simulink model "NPC_inverter_nfE_TS_203864"  (R2023b)
settings: Solver=ode4  StartTime=0.0  StopTime=Tsim  FixedStep=Ts  RelTol=1e-3
InitFcn:
  | run('param_nfE.m');
values from neighbouring files (symbols this model uses):
  f = 50    [param_nfE.m]
  KI = (1/K2)*(1-zR1)*(1-zR1)    [param_nfE.m]
  KP = (1/K2)*(1+K1-2*zR1)    [param_nfE.m]
  LN = 1e-3    (= 0.001)    [param_nfE.m]
  M = (1/K2)*(1-zR1)    [param_nfE.m]
  mmax = 1    [param_nfE.m]
  mmin = -1    [param_nfE.m]
  TA = Tc    (= 0.000125)    [param_nfE.m]
  Tc = 1/fc    (= 0.000125)    [param_nfE.m]
  Umax = Ud/2    (= 350)    [param_nfE.m]
undefined symbols (not defined in the file or in its folder): plecs
libraries: simulink x12, plecslib x5
settings Model: Creator=timsp  LastModifiedBy=timsp

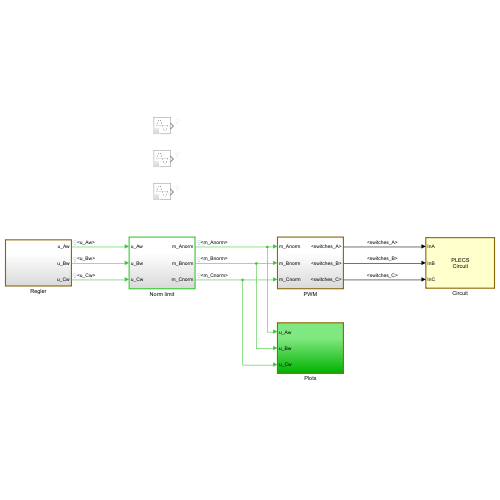
[thumbnail: Simulink's stored preview of the top-level diagram]
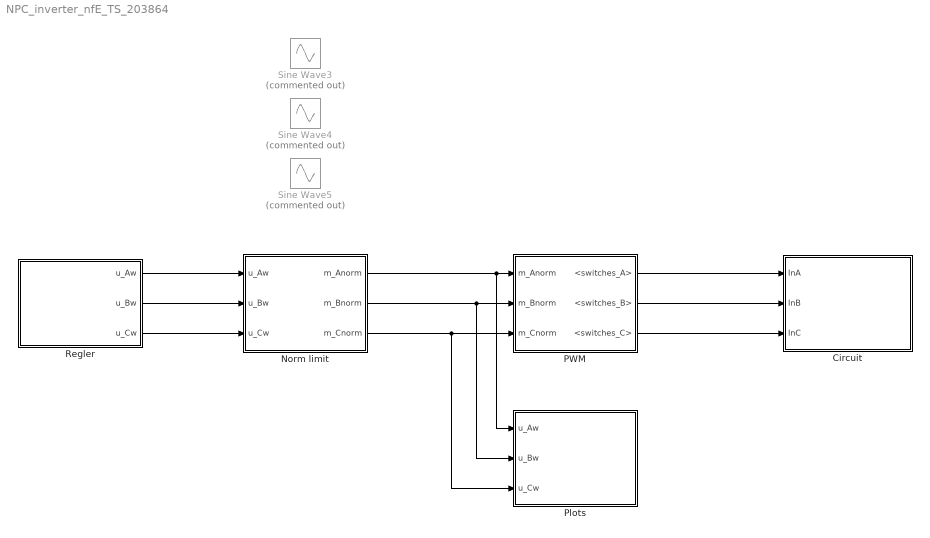
== system NPC_inverter_nfE_TS_203864 ==
  Circuit : Subsystem  LoadFcn=plecs('sl', 200);  InitFcn=plecs('sl', 214);  StartFcn=plecs('sl', 208);  StopFcn=plecs('sl', 209);  mask(PlecsCircuit){PLECSData=<binary blob, 5092 chars, not shown>}
      mask prompts: PLECSData "PLECS Data (Do not delete or modify!)"
      mask init:
      | % PLACE CUSTOM INITIALIZATIONS ABOVE
      | % DO NOT REMOVE
      | plecs('sl', 215);
      | % DO NOT REMOVE
      settings: CopyFcn=plecs('sl', 203);  DeleteFcn=plecs('sl', 205);  UndoDeleteFcn=plecs('sl', 206);  PreSaveFcn=plecs('sl', 211);  PostSaveFcn=plecs('sl', 201);  NameChangeFcn=plecs('sl', 210);  DestroyFcn=plecs('sl', 207);  PreCopyFcn=plecs('sl', 216);  OpenFcn=plecs('sl', 202);  ErrorFcn=plerrorfcn
      mask Help: eval('plecs(''help'', ''qthelp:///creatingacircuit.html'')')
      mask Display: disp('PLECS\nCircuit')
  Norm limit : Subsystem
  PWM : Subsystem
  Plots : Subsystem
  Regler : Subsystem
  Sine Wave3 : Sin  Commented=on  Amplitude=sqrt(2)*230  Frequency=2*pi*f  SampleTime=0
  Sine Wave4 : Sin  Commented=on  Amplitude=sqrt(2)*230  Frequency=2*pi*f  Phase=-2*pi/3  SampleTime=0
  Sine Wave5 : Sin  Commented=on  Amplitude=sqrt(2)*230  Frequency=2*pi*f  Phase=-4*pi/3  SampleTime=0
  wires:
  PWM/1(<switches_A>) -> Circuit/1(InA)
  PWM/2(<switches_B>) -> Circuit/2(InB)
  PWM/3(<switches_C>) -> Circuit/3(InC)
  Norm limit/1(m_Anorm) -> Plots/1(u_Aw), PWM/1(m_Anorm)
  Norm limit/2(m_Bnorm) -> PWM/2(m_Bnorm), Plots/2(u_Bw)
  Norm limit/3(m_Cnorm) -> PWM/3(m_Cnorm), Plots/3(u_Cw)
  Regler/1(u_Aw) -> Norm limit/1(u_Aw)
  Regler/2(u_Bw) -> Norm limit/2(u_Bw)
  Regler/3(u_Cw) -> Norm limit/3(u_Cw)

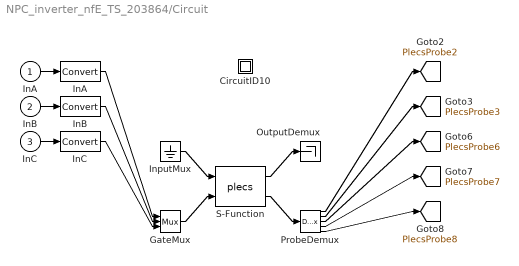
== system NPC_inverter_nfE_TS_203864/Circuit ==
  InA : Inport  PortDimensions=4
  InB : Inport  Port=2  PortDimensions=4
  InC : Inport  Port=3  PortDimensions=4
  " CircuitID10 " : Subsystem
  " GateMux " : Mux  Inputs=[ 4 4 4 ]
  " InA " : DataTypeConversion
  " InB " : DataTypeConversion
  " InC " : DataTypeConversion
  " InputMux " : Ground
  " OutputDemux " : Terminator
  " ProbeDemux " : Demux  Outputs=[ 3 3 3 3 3 ]
  " S-Function " : S-Function  FunctionName=plecs  SFunctionDeploymentMode=off  EnableBusSupport=off
  tag scope: PlecsProbe2=global, PlecsProbe3=global, PlecsProbe6=global, PlecsProbe7=global, PlecsProbe8=global
  wires:
  " InputMux "/1 -> " S-Function "/1
  " GateMux "/1 -> " S-Function "/2
  " S-Function "/1 -> " OutputDemux "/1
  " S-Function "/2 -> " ProbeDemux "/1
  InA/1 -> " InA "/1
  " InA "/1 -> " GateMux "/1
  InB/1 -> " InB "/1
  " InB "/1 -> " GateMux "/2
  InC/1 -> " InC "/1
  " InC "/1 -> " GateMux "/3
  " ProbeDemux "/1 -> [PlecsProbe2]
  " ProbeDemux "/2 -> [PlecsProbe3]
  " ProbeDemux "/3 -> [PlecsProbe6]
  " ProbeDemux "/4 -> [PlecsProbe7]
  " ProbeDemux "/5 -> [PlecsProbe8]

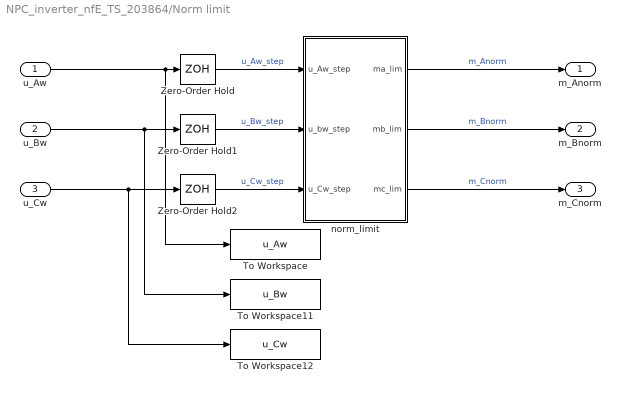
== system NPC_inverter_nfE_TS_203864/Norm limit ==
  u_Aw : Inport
  u_Bw : Inport  Port=2
  u_Cw : Inport  Port=3
  To Workspace : ToWorkspace  VariableName=u_Aw  SampleTime=-1
      settings: Save2DSignal=2-D array (concatenate along first dimension)
  To Workspace11 : ToWorkspace  VariableName=u_Bw  SampleTime=-1
      settings: Save2DSignal=2-D array (concatenate along first dimension)
  To Workspace12 : ToWorkspace  VariableName=u_Cw  SampleTime=-1
      settings: Save2DSignal=2-D array (concatenate along first dimension)
  Zero-Order Hold : ZeroOrderHold  SampleTime=TA
  Zero-Order Hold1 : ZeroOrderHold  SampleTime=TA
  Zero-Order Hold2 : ZeroOrderHold  SampleTime=TA
  norm_limit : Subsystem
  m_Anorm : Outport
  m_Bnorm : Outport  Port=2
  m_Cnorm : Outport  Port=3
  wires:
  norm_limit/2(mb_lim) -> m_Bnorm/1  "m_Bnorm"
  u_Aw/1 -> Zero-Order Hold/1, To Workspace/1
  norm_limit/3(mc_lim) -> m_Cnorm/1  "m_Cnorm"
  Zero-Order Hold1/1 -> norm_limit/2(u_bw_step)  "u_Bw_step"
  u_Bw/1 -> Zero-Order Hold1/1, To Workspace11/1
  Zero-Order Hold/1 -> norm_limit/1(u_Aw_step)  "u_Aw_step"
  u_Cw/1 -> Zero-Order Hold2/1, To Workspace12/1
  Zero-Order Hold2/1 -> norm_limit/3(u_Cw_step)  "u_Cw_step"
  norm_limit/1(ma_lim) -> m_Anorm/1  "m_Anorm"

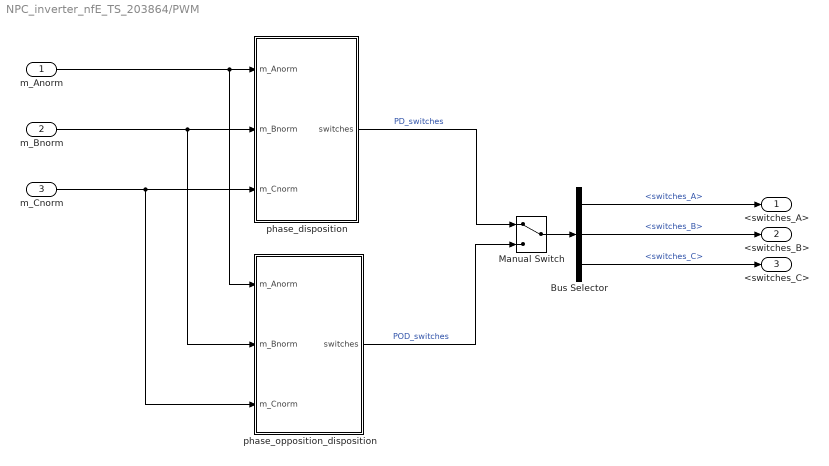
== system NPC_inverter_nfE_TS_203864/PWM ==
  m_Anorm : Inport
  m_Bnorm : Inport  Port=2
  m_Cnorm : Inport  Port=3
  Bus Selector : BusSelector  OutputSignals=switches_A,switches_B,switches_C
  Manual Switch : ManualSwitch
  phase_disposition : Subsystem  TreatAsAtomicUnit=on
  phase_opposition_disposition : Subsystem  TreatAsAtomicUnit=on
  <switches_A> : Outport
  <switches_B> : Outport  Port=2
  <switches_C> : Outport  Port=3
  wires:
  Bus Selector/1 -> <switches_A>/1  "<switches_A>"
  phase_disposition/1(switches) -> Manual Switch/1  "PD_switches"
  Bus Selector/3 -> <switches_C>/1  "<switches_C>"
  phase_opposition_disposition/1(switches) -> Manual Switch/2  "POD_switches"
  Manual Switch/1 -> Bus Selector/1
  Bus Selector/2 -> <switches_B>/1  "<switches_B>"
  m_Anorm/1 -> phase_opposition_disposition/1(m_Anorm), phase_disposition/1(m_Anorm)
  m_Cnorm/1 -> phase_opposition_disposition/3(m_Cnorm), phase_disposition/3(m_Cnorm)
  m_Bnorm/1 -> phase_opposition_disposition/2(m_Bnorm), phase_disposition/2(m_Bnorm)

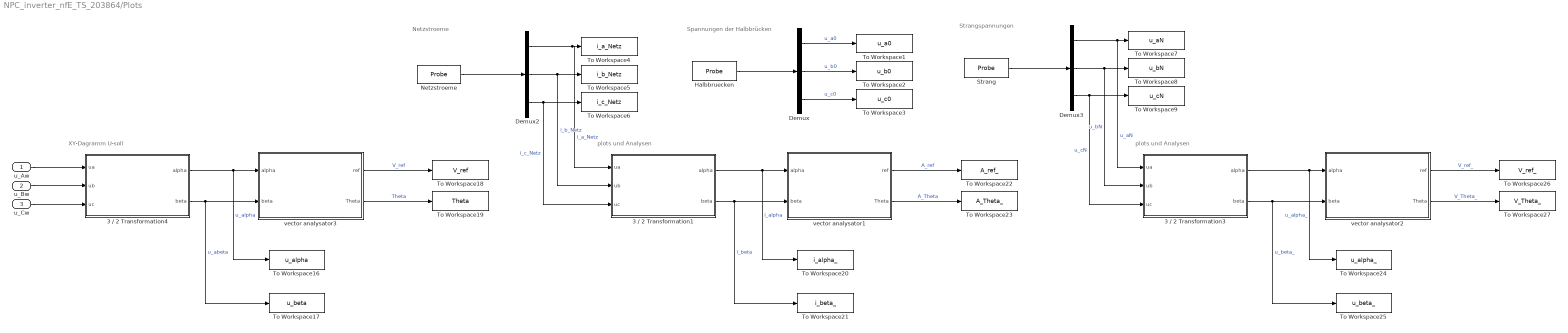
== system NPC_inverter_nfE_TS_203864/Plots ==
  note: Spannungen der Halbbrücken
  note: Strangspannungen
  note: Netzstroeme
  note: plots und Analysen
  note: plots und Analysen
  note: XY-Dagramm U-soll
  u_Aw : Inport
  u_Bw : Inport  Port=2
  u_Cw : Inport  Port=3
  3 / 2 Transformation1 : MATLAB Function  TreatAsAtomicUnit=on
  3 / 2 Transformation3 : MATLAB Function  TreatAsAtomicUnit=on
  3 / 2 Transformation4 : MATLAB Function  TreatAsAtomicUnit=on
  Demux : Demux  Outputs=3
  Demux2 : Demux  Outputs=3
  Demux3 : Demux  Outputs=3
  Halbbruecken : plecslib/Probe  tagno=2
      settings: SourceProductName=PLECS
  Netzstroeme : plecslib/Probe  tagno=8
      settings: SourceProductName=PLECS
  Strang : plecslib/Probe  tagno=3
      settings: SourceProductName=PLECS
  To Workspace1 : ToWorkspace  VariableName=u_a0  SampleTime=-1
  To Workspace16 : ToWorkspace  VariableName=u_alpha  SampleTime=-1
  To Workspace17 : ToWorkspace  VariableName=u_beta  SampleTime=-1
  To Workspace18 : ToWorkspace  VariableName=V_ref  SampleTime=-1
  To Workspace19 : ToWorkspace  VariableName=Theta  SampleTime=-1
  To Workspace2 : ToWorkspace  VariableName=u_b0  SampleTime=-1
  To Workspace20 : ToWorkspace  VariableName=i_alpha_  SampleTime=-1
  To Workspace21 : ToWorkspace  VariableName=i_beta_  SampleTime=-1
  To Workspace22 : ToWorkspace  VariableName=A_ref_  SampleTime=-1
  To Workspace23 : ToWorkspace  VariableName=A_Theta_  SampleTime=-1
  To Workspace24 : ToWorkspace  VariableName=u_alpha_  SampleTime=-1
  To Workspace25 : ToWorkspace  VariableName=u_beta_  SampleTime=-1
  To Workspace26 : ToWorkspace  VariableName=V_ref_  SampleTime=-1
  To Workspace27 : ToWorkspace  VariableName=V_Theta_  SampleTime=-1
  To Workspace3 : ToWorkspace  VariableName=u_c0  SampleTime=-1
  To Workspace4 : ToWorkspace  VariableName=i_a_Netz  SampleTime=-1
  To Workspace5 : ToWorkspace  VariableName=i_b_Netz  SampleTime=-1
  To Workspace6 : ToWorkspace  VariableName=i_c_Netz  SampleTime=-1
  To Workspace7 : ToWorkspace  VariableName=u_aN  SampleTime=-1
  To Workspace8 : ToWorkspace  VariableName=u_bN  SampleTime=-1
  To Workspace9 : ToWorkspace  VariableName=u_cN  SampleTime=-1
  vector analysator1 : MATLAB Function  TreatAsAtomicUnit=on
  vector analysator2 : MATLAB Function  TreatAsAtomicUnit=on
  vector analysator3 : MATLAB Function  TreatAsAtomicUnit=on
  wires:
  Demux2/2 -> To Workspace5/1, 3 / 2 Transformation1/2(ub)  "i_b_Netz"
  Netzstroeme/1 -> Demux2/1
  Demux/3 -> To Workspace3/1  "u_c0"
  3 / 2 Transformation1/2(beta) -> To Workspace21/1, vector analysator1/2(beta)  "i_beta"
  vector analysator2/1(ref) -> To Workspace26/1  "V_ref_"
  3 / 2 Transformation1/1(alpha) -> To Workspace20/1, vector analysator1/1(alpha)  "i_alpha"
  Demux2/1 -> 3 / 2 Transformation1/1(ua), To Workspace4/1  "i_a_Netz"
  3 / 2 Transformation3/2(beta) -> To Workspace25/1, vector analysator2/2(beta)  "u_beta_"
  vector analysator1/2(Theta) -> To Workspace23/1  "A_Theta"
  vector analysator2/2(Theta) -> To Workspace27/1  "V_Theta_"
  3 / 2 Transformation3/1(alpha) -> To Workspace24/1, vector analysator2/1(alpha)  "u_alpha_"
  vector analysator1/1(ref) -> To Workspace22/1  "A_ref"
  Halbbruecken/1 -> Demux/1
  Demux3/1 -> To Workspace7/1, 3 / 2 Transformation3/1(ua)  "u_aN"
  Demux2/3 -> To Workspace6/1, 3 / 2 Transformation1/3(uc)  "i_c_Netz"
  Demux3/3 -> To Workspace9/1, 3 / 2 Transformation3/3(uc)  "u_cN"
  Demux3/2 -> To Workspace8/1, 3 / 2 Transformation3/2(ub)  "u_bN"
  Demux/1 -> To Workspace1/1  "u_a0"
  Strang/1 -> Demux3/1
  Demux/2 -> To Workspace2/1  "u_b0"
  u_Aw/1 -> 3 / 2 Transformation4/1(ua)
  vector analysator3/1(ref) -> To Workspace18/1  "V_ref"
  u_Bw/1 -> 3 / 2 Transformation4/2(ub)
  3 / 2 Transformation4/2(beta) -> To Workspace17/1, vector analysator3/2(beta)  "u_abeta"
  u_Cw/1 -> 3 / 2 Transformation4/3(uc)
  3 / 2 Transformation4/1(alpha) -> To Workspace16/1, vector analysator3/1(alpha)  "u_alpha"
  vector analysator3/2(Theta) -> To Workspace19/1  "Theta"

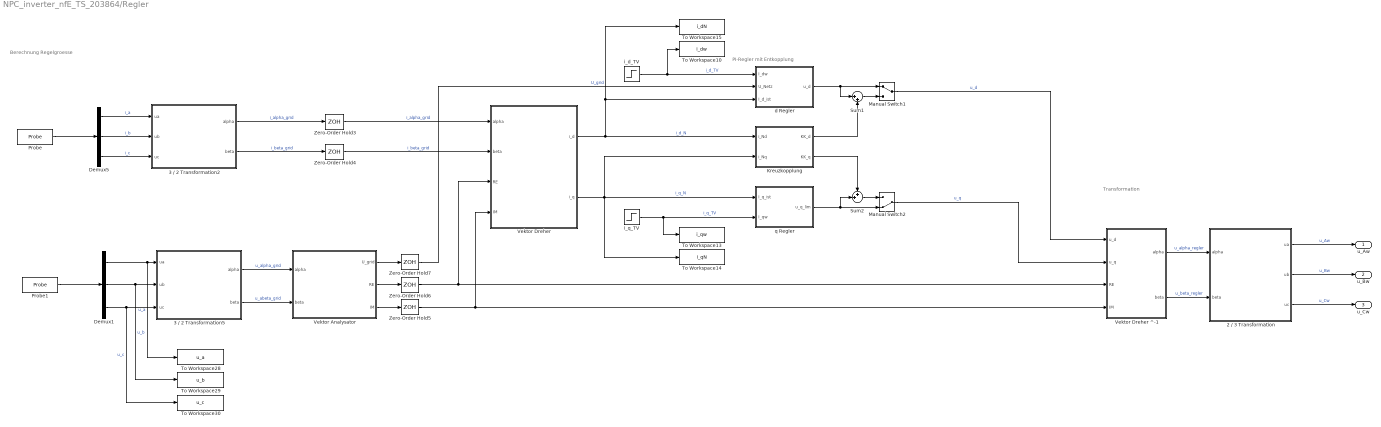
== system NPC_inverter_nfE_TS_203864/Regler ==
  note: Transformation
  note: PI-Regler mit Entkopplung
  note: Berechnung Regelgroesse
  "2 / 3 Transformation " : MATLAB Function  TreatAsAtomicUnit=on
  3 / 2 Transformation2 : MATLAB Function  TreatAsAtomicUnit=on
  3 / 2 Transformation5 : MATLAB Function  TreatAsAtomicUnit=on
  Demux1 : Demux  Outputs=3
  Demux5 : Demux  Outputs=3
  Kreuzkopplung : Subsystem
  Manual Switch1 : ManualSwitch
  Manual Switch2 : ManualSwitch  CurrentSetting=0
  Probe : plecslib/Probe  tagno=6
      settings: SourceProductName=PLECS
  Probe1 : plecslib/Probe  tagno=7
      settings: SourceProductName=PLECS
  Sum1 : Sum  Inputs=|++
  Sum2 : Sum  Inputs=++|
  To Workspace10 : ToWorkspace  VariableName=i_dw  SampleTime=-1
  To Workspace13 : ToWorkspace  VariableName=i_qw  SampleTime=-1
  To Workspace14 : ToWorkspace  VariableName=i_qN  SampleTime=-1
  To Workspace15 : ToWorkspace  VariableName=i_dN  SampleTime=-1
  To Workspace28 : ToWorkspace  VariableName=u_a  SampleTime=-1
  To Workspace29 : ToWorkspace  VariableName=u_b  SampleTime=-1
  To Workspace30 : ToWorkspace  VariableName=u_c  SampleTime=-1
  Vektor Analysator : MATLAB Function  TreatAsAtomicUnit=on
  Vektor Dreher : MATLAB Function  TreatAsAtomicUnit=on
  Vektor Dreher ^-1 : MATLAB Function  TreatAsAtomicUnit=on
  Zero-Order Hold{3..7} (5 alike) : ZeroOrderHold  SampleTime=TA
  d Regler : Subsystem  TreatAsAtomicUnit=on  SystemSampleTime=TA
  i_d_TV : Step  Time=0.025  Before=20  After=-20  SampleTime=TA
  i_q_TV : Step  Time=0.05  After=20  SampleTime=TA
  q Regler : Subsystem  TreatAsAtomicUnit=on  SystemSampleTime=TA
  u_Aw : Outport
  u_Bw : Outport  Port=2
  u_Cw : Outport  Port=3
  wires:
  Vektor Analysator/1(U_grid) -> Zero-Order Hold7/1
  Vektor Dreher/2(i_q) -> Kreuzkopplung/2(i_Nq), q Regler/1(I_q_ist), To Workspace14/1  "i_q_N"
  Vektor Analysator/3(IM) -> Zero-Order Hold5/1
  i_d_TV/1 -> To Workspace10/1, d Regler/1(I_dw)  "i_d_TV"
  Zero-Order Hold4/1 -> Vektor Dreher/2(beta)  "i_beta_grid"
  Zero-Order Hold3/1 -> Vektor Dreher/1(alpha)  "i_alpha_grid"
  Vektor Dreher/1(i_d) -> d Regler/3(I_d_ist), To Workspace15/1, Kreuzkopplung/1(i_Nd)  "i_d_N"
  Probe1/1 -> Demux1/1
  q Regler/1(u_q_lim) -> Manual Switch2/2, Sum2/2
  Manual Switch1/1 -> Vektor Dreher ^-1/1(u_d)  "u_d"
  Sum2/1 -> Manual Switch2/1
  Demux1/1 -> To Workspace28/1, 3 / 2 Transformation5/1(ua)  "u_a"
  Probe/1 -> Demux5/1
  "2 / 3 Transformation "/1(ua) -> u_Aw/1  "u_Aw"
  "2 / 3 Transformation "/3(uc) -> u_Cw/1  "u_Cw"
  3 / 2 Transformation2/2(beta) -> Zero-Order Hold4/1  "i_beta_grid"
  Demux5/1 -> 3 / 2 Transformation2/1(ua)  "i_a"
  i_q_TV/1 -> q Regler/2(I_qw), To Workspace13/1  "i_q_TV"
  Kreuzkopplung/1(KK_d) -> Sum1/2
  Kreuzkopplung/2(KK_q) -> Sum2/1
  Zero-Order Hold5/1 -> Vektor Dreher/4(IM), Vektor Dreher ^-1/4(IM)
  Demux5/2 -> 3 / 2 Transformation2/2(ub)  "i_b"
  Sum1/1 -> Manual Switch1/2
  Zero-Order Hold6/1 -> Vektor Dreher ^-1/3(RE), Vektor Dreher/3(RE)
  Manual Switch2/1 -> Vektor Dreher ^-1/2(u_q)  "u_q"
  Demux5/3 -> 3 / 2 Transformation2/3(uc)  "i_c"
  Vektor Analysator/2(RE) -> Zero-Order Hold6/1
  d Regler/1(u_d) -> Manual Switch1/1, Sum1/1
  Demux1/3 -> To Workspace30/1, 3 / 2 Transformation5/3(uc)  "u_c"
  3 / 2 Transformation2/1(alpha) -> Zero-Order Hold3/1  "i_alpha_grid"
  3 / 2 Transformation5/1(alpha) -> Vektor Analysator/1(alpha)  "u_alpha_grid"
  Demux1/2 -> To Workspace29/1, 3 / 2 Transformation5/2(ub)  "u_b"
  Vektor Dreher ^-1/2(beta) -> "2 / 3 Transformation "/2(beta)  "u_beta_regler"
  3 / 2 Transformation5/2(beta) -> Vektor Analysator/2(beta)  "u_abeta_grid"
  "2 / 3 Transformation "/2(ub) -> u_Bw/1  "u_Bw"
  Zero-Order Hold7/1 -> d Regler/2(U_Netz)  "U_grid"
  Vektor Dreher ^-1/1(alpha) -> "2 / 3 Transformation "/1(alpha)  "u_alpha_regler"

== system NPC_inverter_nfE_TS_203864/Circuit/ CircuitID10  ==

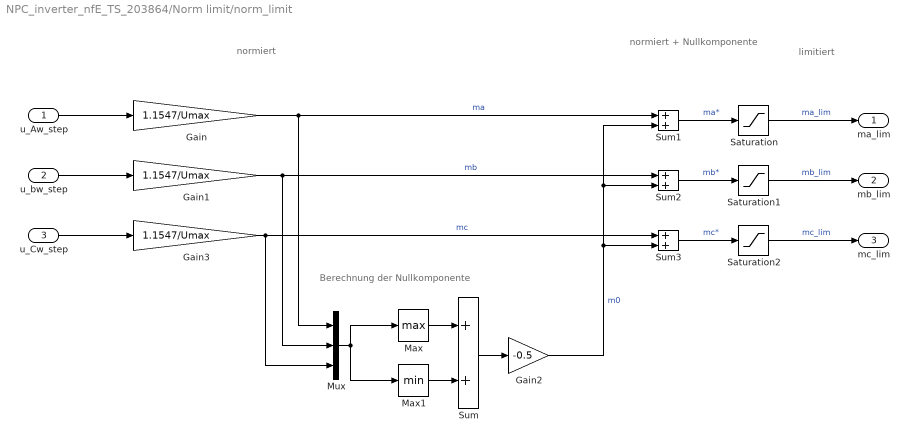
== system NPC_inverter_nfE_TS_203864/Norm limit/norm_limit ==
  note: limitiert
  note: normiert
      | + Nullkomponente
  note: normiert
  note: Berechnung der Nullkomponente
  u_Aw_step : Inport
  u_bw_step : Inport  Port=2
  u_Cw_step : Inport  Port=3
  Gain : Gain  Gain=1.1547/Umax
  Gain1 : Gain  Gain=1.1547/Umax
  Gain2 : Gain  Gain=-0.5
  Gain3 : Gain  Gain=1.1547/Umax
  Max : MinMax  Function=max
  Max1 : MinMax
  Mux : Mux  Inputs=3
  Saturation : Saturate  UpperLimit=mmax  LowerLimit=mmin
  Saturation1 : Saturate  UpperLimit=mmax  LowerLimit=mmin
  Saturation2 : Saturate  UpperLimit=mmax  LowerLimit=mmin
  Sum{,1..3} (4 alike) : Sum
  ma_lim : Outport
  mb_lim : Outport  Port=2
  mc_lim : Outport  Port=3
  wires:
  Gain2/1 -> Sum1/2, Sum2/2, Sum3/2  "m0"
  Sum3/1 -> Saturation2/1  "mc*"
  Sum2/1 -> Saturation1/1  "mb*"
  Sum1/1 -> Saturation/1  "ma*"
  Gain/1 -> Mux/1, Sum1/1  "ma"
  Mux/1 -> Max/1, Max1/1
  Gain1/1 -> Sum2/1, Mux/2  "mb"
  Max1/1 -> Sum/2
  Sum/1 -> Gain2/1
  Max/1 -> Sum/1
  Gain3/1 -> Mux/3, Sum3/1  "mc"
  Saturation2/1 -> mc_lim/1  "mc_lim"
  Saturation1/1 -> mb_lim/1  "mb_lim"
  Saturation/1 -> ma_lim/1  "ma_lim"
  u_Aw_step/1 -> Gain/1
  u_bw_step/1 -> Gain1/1
  u_Cw_step/1 -> Gain3/1

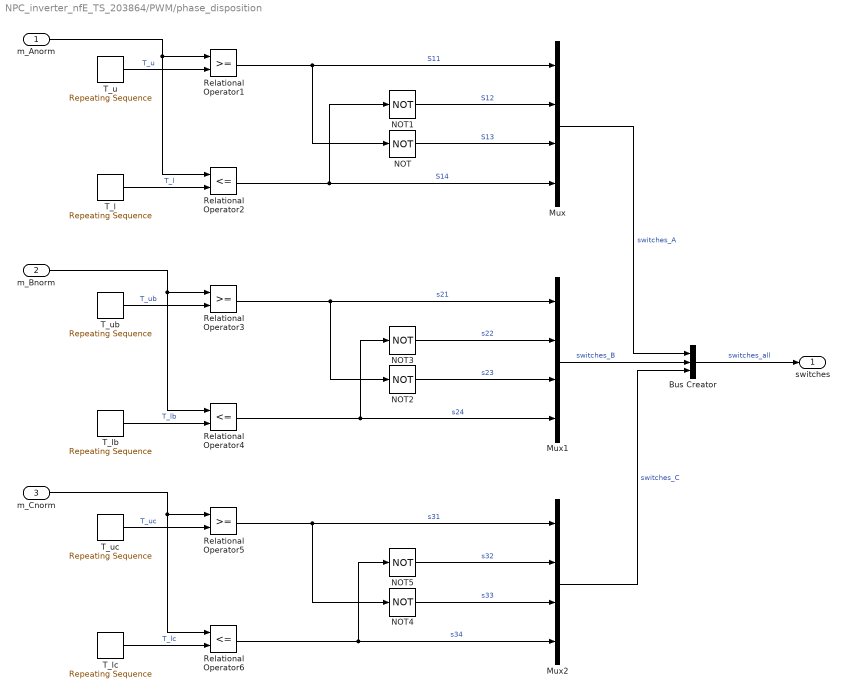
== system NPC_inverter_nfE_TS_203864/PWM/phase_disposition ==
  m_Anorm : Inport
  m_Bnorm : Inport  Port=2
  m_Cnorm : Inport  Port=3
  Bus Creator : BusCreator  Inputs=3
  Mux : Mux
  Mux1 : Mux
  Mux2 : Mux
  NOT{,1..5} (6 alike) : Logic  Operator=NOT  AllPortsSameDT=off  OutDataTypeStr=boolean
  Relational Operator1 : RelationalOperator  OutDataTypeStr=boolean  RndMeth=Simplest  InputSameDT=off
  Relational Operator2 : RelationalOperator  Operator=<=  OutDataTypeStr=boolean  RndMeth=Simplest  InputSameDT=off
  Relational Operator3 : RelationalOperator  OutDataTypeStr=boolean  RndMeth=Simplest  InputSameDT=off
  Relational Operator4 : RelationalOperator  Operator=<=  OutDataTypeStr=boolean  RndMeth=Simplest  InputSameDT=off
  Relational Operator5 : RelationalOperator  OutDataTypeStr=boolean  RndMeth=Simplest  InputSameDT=off
  Relational Operator6 : RelationalOperator  Operator=<=  OutDataTypeStr=boolean  RndMeth=Simplest  InputSameDT=off
  T_l : simulink/Sources/Repeating Sequence  rep_seq_t=[0 Tc/2 Tc]  rep_seq_y=[-1 0 -1]
  T_lb : simulink/Sources/Repeating Sequence  rep_seq_t=[0 Tc/2 Tc]  rep_seq_y=[-1 0 -1]
  T_lc : simulink/Sources/Repeating Sequence  rep_seq_t=[0 Tc/2 Tc]  rep_seq_y=[-1 0 -1]
  T_u : simulink/Sources/Repeating Sequence  rep_seq_t=[0 Tc/2 Tc]  rep_seq_y=[0 1 0]
  T_ub : simulink/Sources/Repeating Sequence  rep_seq_t=[0 Tc/2 Tc]  rep_seq_y=[0 1 0]
  T_uc : simulink/Sources/Repeating Sequence  rep_seq_t=[0 Tc/2 Tc]  rep_seq_y=[0 1 0]
  switches : Outport
  wires:
  Bus Creator/1 -> switches/1  "switches_all"
  m_Anorm/1 -> Relational Operator2/1, Relational Operator1/1
  Relational Operator1/1 -> NOT/1, Mux/1  "S11"
  Relational Operator2/1 -> NOT1/1, Mux/4  "S14"
  T_l/1 -> Relational Operator2/2  "T_l"
  T_u/1 -> Relational Operator1/2  "T_u"
  NOT/1 -> Mux/3  "S13"
  NOT1/1 -> Mux/2  "S12"
  NOT2/1 -> Mux1/3  "s23"
  NOT3/1 -> Mux1/2  "s22"
  T_lb/1 -> Relational Operator4/2  "T_lb"
  Relational Operator3/1 -> NOT2/1, Mux1/1  "s21"
  Relational Operator4/1 -> Mux1/4, NOT3/1  "s24"
  T_ub/1 -> Relational Operator3/2  "T_ub"
  T_uc/1 -> Relational Operator5/2  "T_uc"
  Relational Operator6/1 -> Mux2/4, NOT5/1  "s34"
  T_lc/1 -> Relational Operator6/2  "T_lc"
  NOT4/1 -> Mux2/3  "s33"
  Relational Operator5/1 -> NOT4/1, Mux2/1  "s31"
  NOT5/1 -> Mux2/2  "s32"
  Mux/1 -> Bus Creator/1  "switches_A"
  Mux1/1 -> Bus Creator/2  "switches_B"
  Mux2/1 -> Bus Creator/3  "switches_C"
  m_Cnorm/1 -> Relational Operator6/1, Relational Operator5/1
  m_Bnorm/1 -> Relational Operator4/1, Relational Operator3/1

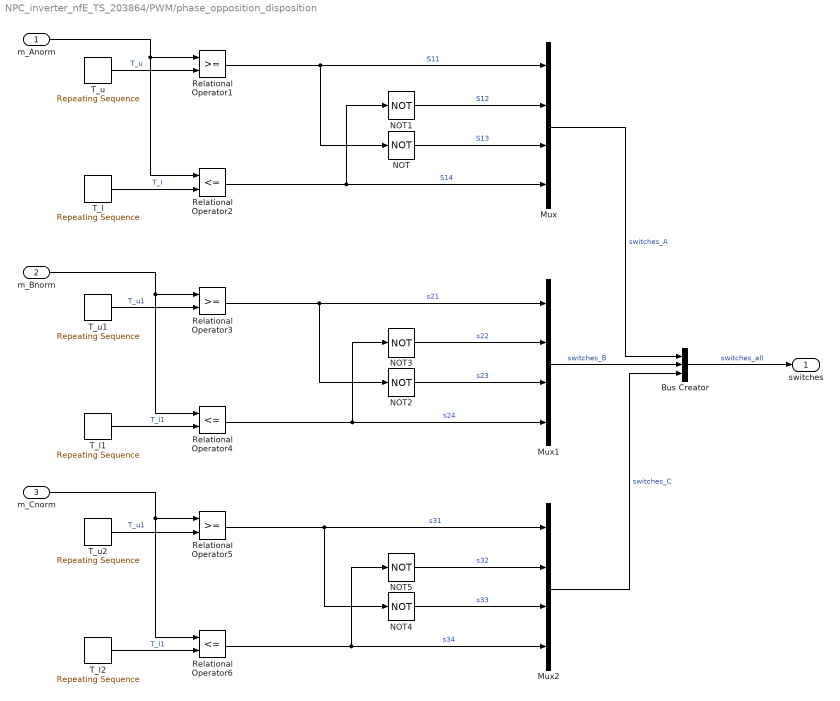
== system NPC_inverter_nfE_TS_203864/PWM/phase_opposition_disposition ==
  m_Anorm : Inport
  m_Bnorm : Inport  Port=2
  m_Cnorm : Inport  Port=3
  Bus Creator : BusCreator  Inputs=3
  Mux : Mux
  Mux1 : Mux
  Mux2 : Mux
  NOT{,1..5} (6 alike) : Logic  Operator=NOT  AllPortsSameDT=off  OutDataTypeStr=boolean
  Relational Operator1 : RelationalOperator  OutDataTypeStr=boolean  RndMeth=Simplest  InputSameDT=off
  Relational Operator2 : RelationalOperator  Operator=<=  OutDataTypeStr=boolean  RndMeth=Simplest  InputSameDT=off
  Relational Operator3 : RelationalOperator  OutDataTypeStr=boolean  RndMeth=Simplest  InputSameDT=off
  Relational Operator4 : RelationalOperator  Operator=<=  OutDataTypeStr=boolean  RndMeth=Simplest  InputSameDT=off
  Relational Operator5 : RelationalOperator  OutDataTypeStr=boolean  RndMeth=Simplest  InputSameDT=off
  Relational Operator6 : RelationalOperator  Operator=<=  OutDataTypeStr=boolean  RndMeth=Simplest  InputSameDT=off
  T_l : simulink/Sources/Repeating Sequence  rep_seq_t=[0 Tc/2 Tc]  rep_seq_y=[ 0 -1 0]
  T_l1 : simulink/Sources/Repeating Sequence  rep_seq_t=[0 Tc/2 Tc]  rep_seq_y=[0 -1 0]
  T_l2 : simulink/Sources/Repeating Sequence  rep_seq_t=[0 Tc/2 Tc]  rep_seq_y=[0 -1 0]
  T_u : simulink/Sources/Repeating Sequence  rep_seq_t=[0 Tc/2 Tc]  rep_seq_y=[0 1 0]
  T_u1 : simulink/Sources/Repeating Sequence  rep_seq_t=[0 Tc/2 Tc]  rep_seq_y=[0 1 0]
  T_u2 : simulink/Sources/Repeating Sequence  rep_seq_t=[0 Tc/2 Tc]  rep_seq_y=[0 1 0]
  switches : Outport
  wires:
  Relational Operator6/1 -> NOT5/1, Mux2/4  "s34"
  Bus Creator/1 -> switches/1  "switches_all"
  Relational Operator3/1 -> NOT2/1, Mux1/1  "s21"
  m_Anorm/1 -> Relational Operator2/1, Relational Operator1/1
  T_u/1 -> Relational Operator1/2  "T_u"
  T_l/1 -> Relational Operator2/2  "T_l"
  NOT2/1 -> Mux1/3  "s23"
  Relational Operator1/1 -> Mux/1, NOT/1  "S11"
  Relational Operator2/1 -> Mux/4, NOT1/1  "S14"
  NOT1/1 -> Mux/2  "S12"
  Mux2/1 -> Bus Creator/3  "switches_C"
  NOT3/1 -> Mux1/2  "s22"
  NOT4/1 -> Mux2/3  "s33"
  m_Bnorm/1 -> Relational Operator4/1, Relational Operator3/1
  NOT5/1 -> Mux2/2  "s32"
  T_u2/1 -> Relational Operator5/2  "T_u1"
  Mux1/1 -> Bus Creator/2  "switches_B"
  NOT/1 -> Mux/3  "S13"
  Relational Operator4/1 -> NOT3/1, Mux1/4  "s24"
  Relational Operator5/1 -> Mux2/1, NOT4/1  "s31"
  T_u1/1 -> Relational Operator3/2  "T_u1"
  Mux/1 -> Bus Creator/1  "switches_A"
  T_l1/1 -> Relational Operator4/2  "T_l1"
  m_Cnorm/1 -> Relational Operator6/1, Relational Operator5/1
  T_l2/1 -> Relational Operator6/2  "T_l1"

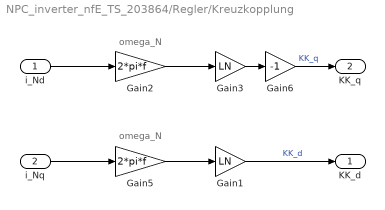
== system NPC_inverter_nfE_TS_203864/Regler/Kreuzkopplung ==
  note: omega_N
  note: omega_N
  i_Nd : Inport
  i_Nq : Inport  Port=2
  Gain1 : Gain  Gain=LN
  Gain2 : Gain  Gain=2*pi*f
  Gain3 : Gain  Gain=LN
  Gain5 : Gain  Gain=2*pi*f
  Gain6 : Gain  Gain=-1
  KK_d : Outport
  KK_q : Outport  Port=2
  wires:
  Gain1/1 -> KK_d/1  "KK_d"
  Gain3/1 -> Gain6/1
  Gain2/1 -> Gain3/1
  i_Nd/1 -> Gain2/1
  Gain5/1 -> Gain1/1
  i_Nq/1 -> Gain5/1
  Gain6/1 -> KK_q/1  "KK_q"

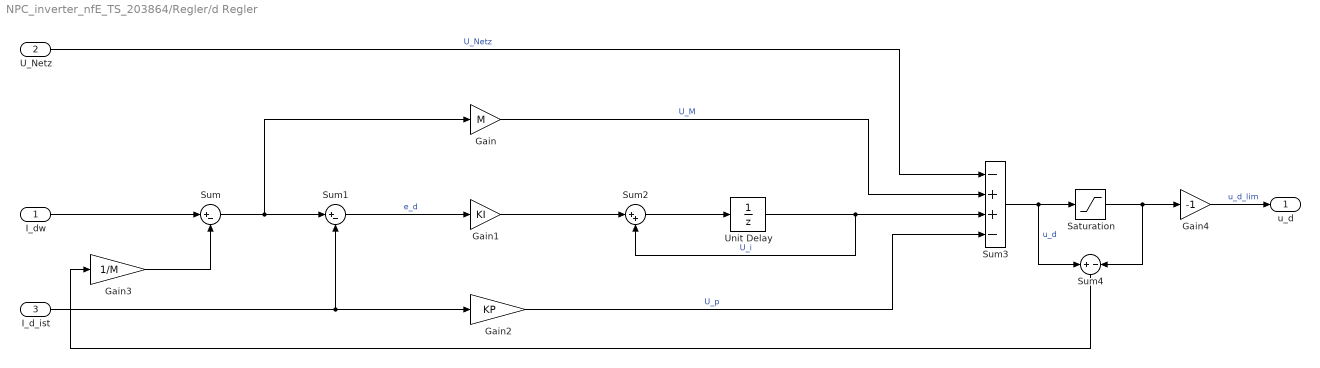
== system NPC_inverter_nfE_TS_203864/Regler/d Regler ==
  I_dw : Inport
  U_Netz : Inport  Port=2
  I_d_ist : Inport  Port=3
  Gain : Gain  Gain=M
  Gain1 : Gain  Gain=KI
  Gain2 : Gain  Gain=KP
  Gain3 : Gain  Gain=1/M
  Gain4 : Gain  Gain=-1
  Saturation : Saturate  UpperLimit=mmax*Umax  LowerLimit=mmin*Umax
  Sum : Sum  Inputs=|+-
  Sum1 : Sum  Inputs=|+-
  Sum2 : Sum  Inputs=|++
  Sum3 : Sum  Inputs=-++-
  Sum4 : Sum  Inputs=+|-
  Unit Delay : UnitDelay  SampleTime=TA  HasFrameUpgradeWarning=on
  u_d : Outport
  wires:
  U_Netz/1 -> Sum3/1  "U_Netz"
  Sum4/1 -> Gain3/1
  Gain3/1 -> Sum/2
  Gain2/1 -> Sum3/4  "U_p"
  Gain/1 -> Sum3/2  "U_M"
  Sum3/1 -> Saturation/1, Sum4/1  "u_d"
  Saturation/1 -> Gain4/1, Sum4/2
  Unit Delay/1 -> Sum3/3, Sum2/2  "U_i"
  Sum2/1 -> Unit Delay/1
  Gain1/1 -> Sum2/1
  Sum1/1 -> Gain1/1  "e_d"
  Sum/1 -> Sum1/1, Gain/1
  I_d_ist/1 -> Sum1/2, Gain2/1
  I_dw/1 -> Sum/1
  Gain4/1 -> u_d/1  "u_d_lim"

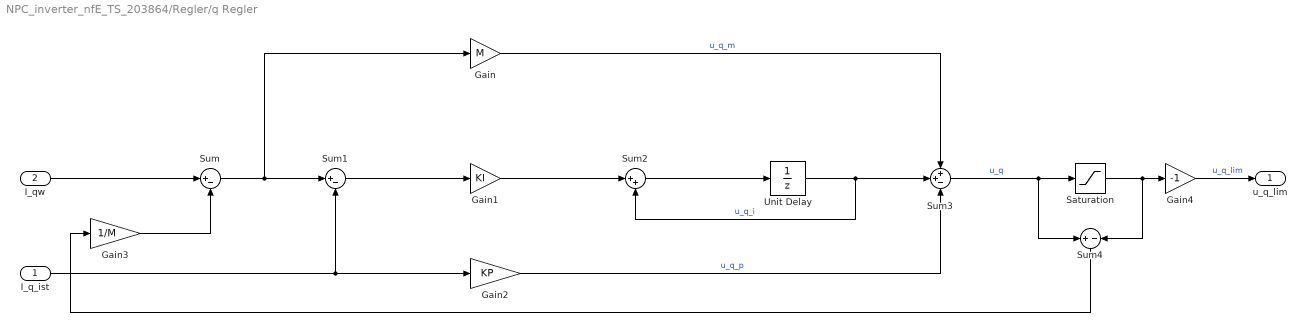
== system NPC_inverter_nfE_TS_203864/Regler/q Regler ==
  I_q_ist : Inport
  I_qw : Inport  Port=2
  Gain : Gain  Gain=M
  Gain1 : Gain  Gain=KI
  Gain2 : Gain  Gain=KP
  Gain3 : Gain  Gain=1/M
  Gain4 : Gain  Gain=-1
  Saturation : Saturate  UpperLimit=mmax*Umax  LowerLimit=mmin*Umax
  Sum : Sum  Inputs=|+-
  Sum1 : Sum  Inputs=|+-
  Sum2 : Sum  Inputs=|++
  Sum3 : Sum  Inputs=++-
  Sum4 : Sum  Inputs=+|-
  Unit Delay : UnitDelay  SampleTime=TA  HasFrameUpgradeWarning=on
  u_q_lim : Outport
  wires:
  Sum/1 -> Sum1/1, Gain/1
  Sum2/1 -> Unit Delay/1
  Gain/1 -> Sum3/1  "u_q_m"
  Gain3/1 -> Sum/2
  Saturation/1 -> Gain4/1, Sum4/2
  I_q_ist/1 -> Sum1/2, Gain2/1
  I_qw/1 -> Sum/1
  Gain1/1 -> Sum2/1
  Gain2/1 -> Sum3/3  "u_q_p"
  Unit Delay/1 -> Sum2/2, Sum3/2  "u_q_i"
  Sum4/1 -> Gain3/1
  Sum3/1 -> Saturation/1, Sum4/1  "u_q"
  Sum1/1 -> Gain1/1
  Gain4/1 -> u_q_lim/1  "u_q_lim"

== matlab function NPC_inverter_nfE_TS_203864/Regler/Vektor Analysator ==
  data: U_grid output; RE output; IM output; alpha input; beta input
function [U_grid, RE, IM]= fcn(alpha, beta)


    U_grid = sqrt(alpha^2+beta^2);

    %Theta = atan2(beta, alpha); % damit Theta [0, 2pi]

    RE = alpha/U_grid;
    
    IM = beta/U_grid;

end

== matlab function NPC_inverter_nfE_TS_203864/Regler/Vektor Dreher ==
  data: alpha input; i_d output; beta input; RE input; IM input; i_q output
function [i_d, i_q]= fcn(alpha, beta, RE, IM)


    
    z = [alpha; beta];

    T =[RE IM ;...
        -IM RE];

    y = T * z;    % [i_alpha ; i_beta]

    i_d = y(1);
    i_q = y(2);

end

== matlab function NPC_inverter_nfE_TS_203864/Regler/Vektor Dreher ^-1 ==
  data: u_d input; alpha output; u_q input; RE input; IM input; beta output
function [alpha, beta] = fcn(u_d, u_q, RE, IM)
    
    z = [u_d;u_q];

    T =[RE -IM ;...
        IM RE];

    y = T * z;    % [alpha; beta]
    
    alpha = y(1);
    beta = y(2);
    %out_0 = 0;

end

== matlab function NPC_inverter_nfE_TS_203864/Plots/vector analysator3 ==
  data: alpha input; ref output; Theta output; beta input
function [ref, Theta]= fcn(alpha, beta)
% ### input vector ###
% u1 = alpha (real part or space vector)
% u2 = beta (imaginary part of space vector)

% ### output vector ###
% y1 = ref (absolute value)
% y2 = Theta (angle)

% ### calculation ####
    ref = sqrt(alpha^2+beta^2);

    Theta = atan2(beta, alpha); % damit Theta [0, 2pi]

end

== matlab function NPC_inverter_nfE_TS_203864/Plots/3 // 2 Transformation1 ==
  data: ua input; alpha output; ub input; uc input; beta output
function [alpha, beta] = fcn(ua, ub, uc)
% ### input vector ###
% u1 = ua
% u2 = ub
% u3 = uc

% ### output vector ###
% y1 = alpha
% y2 = beta
% y3 = u_0

% ### calculation ###
    T = 2/3.*   [1 -1/2 -1/2;...
                0 sqrt(3)/2 -sqrt(3)/2;...
                1/2 1/2 1/2];
    
    y = T * [ua; ub; uc];   
    
% ### return ###
    alpha = y(1);
    beta = y(2);
    %u_0 = y(3);
end

== matlab function NPC_inverter_nfE_TS_203864/Plots/vector analysator1 ==
  data: alpha input; ref output; Theta output; beta input
function [ref, Theta]= fcn(alpha, beta)
% ### input vector ###
% u1 = alpha (real part or space vector)
% u2 = beta (imaginary part of space vector)

% ### output vector ###
% y1 = ref (absolute value)
% y2 = Theta (angle)

% ### calculation ####
    ref = sqrt(alpha^2+beta^2);

    Theta = atan2(beta, alpha); % damit Theta [0, 2pi]

end

== matlab function NPC_inverter_nfE_TS_203864/Plots/3 // 2 Transformation3 ==
  data: ua input; alpha output; ub input; uc input; beta output
function [alpha, beta] = fcn(ua, ub, uc)
% ### input vector ###
% u1 = ua
% u2 = ub
% u3 = uc

% ### output vector ###
% y1 = alpha
% y2 = beta
% y3 = u_0

% ### calculation ###
    T = 2/3.*   [1 -1/2 -1/2;...
                0 sqrt(3)/2 -sqrt(3)/2;...
                1/2 1/2 1/2];
    
    y = T * [ua; ub; uc];   
    
% ### return ###
    alpha = y(1);
    beta = y(2);
    %u_0 = y(3);
end

== matlab function NPC_inverter_nfE_TS_203864/Plots/3 // 2 Transformation4 ==
  data: ua input; alpha output; ub input; uc input; beta output
function [alpha, beta] = fcn(ua, ub, uc)
% ### input vector ###
% u1 = ua
% u2 = ub
% u3 = uc

% ### output vector ###
% y1 = alpha
% y2 = beta
% y3 = u_0

% ### calculation ###
    T = 2/3.*   [1 -1/2 -1/2;...
                0 sqrt(3)/2 -sqrt(3)/2;...
                1/2 1/2 1/2];
    
    y = T * [ua; ub; uc];   
    
% ### return ###
    alpha = y(1);
    beta = y(2);
    %u_0 = y(3);
end

== matlab function NPC_inverter_nfE_TS_203864/Plots/vector analysator2 ==
  data: alpha input; ref output; Theta output; beta input
function [ref, Theta]= fcn(alpha, beta)
% ### input vector ###
% u1 = alpha (real part or space vector)
% u2 = beta (imaginary part of space vector)

% ### output vector ###
% y1 = ref (absolute value)
% y2 = Theta (angle)

% ### calculation ####
    ref = sqrt(alpha^2+beta^2);

    Theta = atan2(beta, alpha); % damit Theta [0, 2pi]

end

== matlab function NPC_inverter_nfE_TS_203864/Regler/2 // 3 Transformation  ==
  data: alpha input; ua output; beta input; ub output; uc output
function [ua, ub, uc] = fcn(alpha, beta)
% ### input vector ###
% y1 = alpha
% y2 = beta
% y3 = u_0 --> no actual input

% ### output vector ###
% u1 = ua
% u2 = ub
% u3 = uc

% ### calculation ###

    T =    [1      0         1;...
           -1/2  sqrt(3)/2   1;...
           -1/2 -sqrt(3)/2   1];
    
    y = T * [alpha; beta; 0];   

% ### return ###
    ua = y(1);
    ub = y(2);
    uc = y(3);
end

== matlab function NPC_inverter_nfE_TS_203864/Regler/3 // 2 Transformation2 ==
  data: ua input; alpha output; ub input; uc input; beta output
function [alpha, beta] = fcn(ua, ub, uc)
% ### input vector ###
% u1 = ua
% u2 = ub
% u3 = uc

% ### output vector ###
% y1 = alpha
% y2 = beta
% y3 = u_0

% ### calculation ###
    T = 2/3.*   [1 -1/2 -1/2;...
                0 sqrt(3)/2 -sqrt(3)/2;...
                1/2 1/2 1/2];
    
    y = T * [ua; ub; uc];   
    
% ### return ###
    alpha = y(1);
    beta = y(2);
    %u_0 = y(3);
end

== matlab function NPC_inverter_nfE_TS_203864/Regler/3 // 2 Transformation5 ==
  data: ua input; alpha output; ub input; uc input; beta output
function [alpha, beta] = fcn(ua, ub, uc)
% ### input vector ###
% u1 = ua
% u2 = ub
% u3 = uc

% ### output vector ###
% y1 = alpha
% y2 = beta
% y3 = u_0

% ### calculation ###
    T = 2/3.*   [1 -1/2 -1/2;...
                0 sqrt(3)/2 -sqrt(3)/2;...
                1/2 1/2 1/2];
    
    y = T * [ua; ub; uc];   
    
% ### return ###
    alpha = y(1);
    beta = y(2);
    %u_0 = y(3);
end
